simulink library "GTPR_Library"  (R2021a)
settings: Solver=VariableStepAuto  StartTime=0.0  StopTime=10.0  RelTol=1e-3
values from neighbouring files (symbols this model uses):
  aA = 0.5    [SimMechanics_GTPR_OpenLoop_CircularMotion_VS_ClosedLoop.m]
  aB = 0.5    [SimMechanics_GTPR_OpenLoop_CircularMotion_VS_ClosedLoop.m]
  aC = 0.5    [SimMechanics_GTPR_OpenLoop_CircularMotion_VS_ClosedLoop.m]
  alphaAB = deg2rad(120)    [SimMechanics_GTPR_OpenLoop_CircularMotion_VS_ClosedLoop.m]
  alphaAC = deg2rad(240)    [SimMechanics_GTPR_OpenLoop_CircularMotion_VS_ClosedLoop.m]
  eA = 0.28    [SimMechanics_GTPR_OpenLoop_CircularMotion_VS_ClosedLoop.m]
  eB = 0.28    [SimMechanics_GTPR_OpenLoop_CircularMotion_VS_ClosedLoop.m]
  eC = 0.28    [SimMechanics_GTPR_OpenLoop_CircularMotion_VS_ClosedLoop.m]
  g = -9.81    [SimMechanics_GTPR_OpenLoop_CircularMotion_VS_ClosedLoop.m]
  ILA = zeros(3)    [SimMechanics_GTPR_OpenLoop_CircularMotion_VS_ClosedLoop.m]
  IlA = zeros(3)    [SimMechanics_GTPR_OpenLoop_CircularMotion_VS_ClosedLoop.m]
  ILB = zeros(3)    [SimMechanics_GTPR_OpenLoop_CircularMotion_VS_ClosedLoop.m]
  IlB = zeros(3)    [SimMechanics_GTPR_OpenLoop_CircularMotion_VS_ClosedLoop.m]
  ILC = zeros(3)    [SimMechanics_GTPR_OpenLoop_CircularMotion_VS_ClosedLoop.m]
  IlC = zeros(3)    [SimMechanics_GTPR_OpenLoop_CircularMotion_VS_ClosedLoop.m]
  LA = 0.57    [SimMechanics_GTPR_OpenLoop_CircularMotion_VS_ClosedLoop.m]
  lA = 0.9    [SimMechanics_GTPR_OpenLoop_CircularMotion_VS_ClosedLoop.m]
  LB = 0.57    [SimMechanics_GTPR_OpenLoop_CircularMotion_VS_ClosedLoop.m]
  lB = 0.9    [SimMechanics_GTPR_OpenLoop_CircularMotion_VS_ClosedLoop.m]
  LC = 0.57    [SimMechanics_GTPR_OpenLoop_CircularMotion_VS_ClosedLoop.m]
  lC = 0.9    [SimMechanics_GTPR_OpenLoop_CircularMotion_VS_ClosedLoop.m]
  m_unaccounted = 1e-16    [SimMechanics_GTPR_OpenLoop_CircularMotion_VS_ClosedLoop.m]
  mLA = density_upperArm*VLA    (= 1.4415197891)    [SimMechanics_GTPR_OpenLoop_CircularMotion_VS_ClosedLoop.m]
  mlA = density_LowerArm*VlA    (= 0.190851753706)    [SimMechanics_GTPR_OpenLoop_CircularMotion_VS_ClosedLoop.m]
  mLB = density_upperArm*VLB    (= 1.4415197891)    [SimMechanics_GTPR_OpenLoop_CircularMotion_VS_ClosedLoop.m]
  mlB = density_LowerArm*VlB    (= 0.190851753706)    [SimMechanics_GTPR_OpenLoop_CircularMotion_VS_ClosedLoop.m]
  mLC = density_upperArm*VLC    (= 1.4415197891)    [SimMechanics_GTPR_OpenLoop_CircularMotion_VS_ClosedLoop.m]
  mlC = density_LowerArm*VlC    (= 0.190851753706)    [SimMechanics_GTPR_OpenLoop_CircularMotion_VS_ClosedLoop.m]
  mTCP = density_workTriangle * VTCP    [SimMechanics_GTPR_OpenLoop_CircularMotion_VS_ClosedLoop.m]
undefined symbols (not defined in the file or in its folder): dq1, dq2, dq3, q1, q2, q3, X, Y, Z
libraries: sm_lib x83, $bdroot x31, nesl_utility x24
(part 4 of 8)

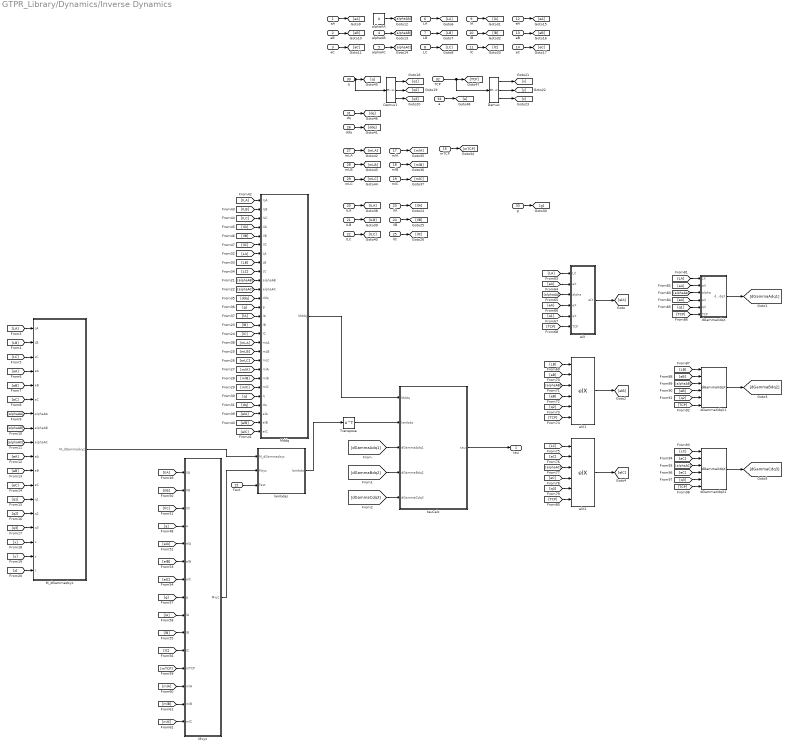
== system GTPR_Library/Dynamics/Inverse Dynamics ==
  aA : Inport
  aB : Inport  Port=2
  aC : Inport  Port=3
  alphaAB : Inport  Port=4
  alphaAC : Inport  Port=5
  LA : Inport  Port=6
  LB : Inport  Port=7
  LC : Inport  Port=8
  lA : Inport  Port=9
  lB : Inport  Port=10
  lC : Inport  Port=11
  eA : Inport  Port=12
  eB : Inport  Port=13
  eC : Inport  Port=14
  Fext : Inport  Port=15
  mTCP : Inport  Port=16
  mlA : Inport  Port=17
  mlB : Inport  Port=18
  mlC : Inport  Port=19
  ILA : Inport  Port=20
  ILB : Inport  Port=21
  ILC : Inport  Port=22
  IlA : Inport  Port=23
  IlB : Inport  Port=24
  IlC : Inport  Port=25
  ddq : Inport  Port=26
  mLA : Inport  Port=27
  mLB : Inport  Port=28
  mLC : Inport  Port=29
  q : Inport  Port=30
  dq : Inport  Port=31
  TCP : Inport  Port=32
  g : Inport  Port=33
  a : Inport  Port=34
  Demux : Demux  Outputs=3
  Demux1 : Demux  Outputs=3
  M_dGammadxyz : Subsystem
  Mddq : Subsystem
  Mxyz : Subsystem
  Transpose : Math  Operator=transpose  SaturateOnIntegerOverflow=on
  alphaAA : Constant  Value=0
  dGammaXdqX : Subsystem
  dGammaXdqX1 : $bdroot/Dynamics/Inverse Dynamics/dGammaXdqX  SystemSampleTime=-1  VariantActivationTime=update diagram  Latency=0  AutoFrameSizeCalculation=off
  dGammaXdqX2 : $bdroot/Dynamics/Inverse Dynamics/dGammaXdqX  SystemSampleTime=-1  VariantActivationTime=update diagram  Latency=0  AutoFrameSizeCalculation=off
  elX : Subsystem
  elX1 : $bdroot/Dynamics/Inverse Dynamics/elX  SystemSampleTime=-1  VariantActivationTime=update diagram  Latency=0  AutoFrameSizeCalculation=off
  elX2 : $bdroot/Dynamics/Inverse Dynamics/elX  SystemSampleTime=-1  VariantActivationTime=update diagram  Latency=0  AutoFrameSizeCalculation=off
  lambdas : MATLAB Function  TreatAsAtomicUnit=on
  tauCalc : MATLAB Function  TreatAsAtomicUnit=on
  tau : Outport
  wires:
  M_dGammadxyz/1(M_dGammadxyz) -> lambdas/1(M_dGammadxyz)
  Mxyz/1(Mxyz) -> lambdas/2(Mxyz)
  Fext/1 -> lambdas/3(Fext)
  Mddq/1(Mddq) -> tauCalc/1(Mddq)
  lambdas/1(lambda) -> Transpose/1
  elX/1(elX) -> [elA]
  dGammaXdqX/1(dGammaXdqX) -> [dGammaAdq1]
  dGammaXdqX1/1 -> [dGammaBdq2]
  elX1/1 -> [elB]
  dGammaXdqX2/1 -> [dGammaCdq3]
  elX2/1 -> [elC]
  [dGammaAdq1] -> tauCalc/3(dGammaAdq1)
  [dGammaBdq2] -> tauCalc/4(dGammaBdq2)
  [dGammaCdq3] -> tauCalc/5(dGammaCdq3)
  tauCalc/1(tau) -> tau/1
  LA/1 -> [LA]
  LB/1 -> [LB]
  LC/1 -> [LC]
  aA/1 -> [aA]
  aB/1 -> [aB]
  aC/1 -> [aC]
  alphaAA/1 -> [alphaAA]
  alphaAB/1 -> [alphaAB]
  alphaAC/1 -> [alphaAC]
  mTCP/1 -> [mTCP]
  mlA/1 -> [mlA]
  mlB/1 -> [mlB]
  mlC/1 -> [mlC]
  ILA/1 -> [ILA]
  ILB/1 -> [ILB]
  ILC/1 -> [ILC]
  ddq/1 -> [ddq]
  mLA/1 -> [mLA]
  mLB/1 -> [mLB]
  mLC/1 -> [mLC]
  q/1 -> Demux1/1, [q]
  dq/1 -> [dq]
  TCP/1 -> Demux/1, [TCP]
  lA/1 -> [lA]
  lB/1 -> [lB]
  lC/1 -> [lC]
  eC/1 -> [eC]
  eB/1 -> [eB]
  eA/1 -> [eA]
  Demux/1 -> [x]
  Demux/2 -> [y]
  Demux/3 -> [z]
  IlB/1 -> [IlB]
  g/1 -> [g]
  IlC/1 -> [IlC]
  IlA/1 -> [IlA]
  Demux1/2 -> [q2]
  Demux1/1 -> [q1]
  Demux1/3 -> [q3]
  [LA] -> M_dGammadxyz/1(LA)
  [LB] -> M_dGammadxyz/2(LB)
  [LC] -> M_dGammadxyz/3(LC)
  [aA] -> M_dGammadxyz/4(aA)
  [aB] -> M_dGammadxyz/5(aB)
  [aC] -> M_dGammadxyz/6(aC)
  [alphaAA] -> M_dGammadxyz/7(alphaAA)
  [alphaAB] -> M_dGammadxyz/8(alphaAB)
  [alphaAC] -> M_dGammadxyz/9(alphaAC)
  [eA] -> M_dGammadxyz/10(eA)
  [eB] -> M_dGammadxyz/11(eB)
  [eC] -> M_dGammadxyz/12(eC)
  [q1] -> M_dGammadxyz/13(q1)
  [q2] -> M_dGammadxyz/14(q2)
  [q3] -> M_dGammadxyz/15(q3)
  [x] -> M_dGammadxyz/16(x)
  [y] -> M_dGammadxyz/17(y)
  [z] -> M_dGammadxyz/18(z)
  [mLA] -> Mddq/17(mLA)
  [lB] -> Mddq/15(lB)
  [mLB] -> Mddq/18(mLB)
  [LA] -> Mddq/7(LA)
  [q] -> Mddq/23(q)
  [alphaAC] -> Mddq/11(alphaAC)
  [ddq] -> Mddq/12(ddq)
  [dq] -> Mddq/24(dq)
  [lC] -> Mddq/16(lC)
  [alphaAB] -> Mddq/10(alphaAB)
  [mLC] -> Mddq/19(mLC)
  [lA] -> Mddq/14(lA)
  [LB] -> Mddq/8(LB)
  [mlB] -> Mddq/21(mlB)
  [mlA] -> Mddq/20(mlA)
  [g] -> Mddq/13(g)
  [LC] -> Mddq/9(LC)
  [mlC] -> Mddq/22(mlC)
  [elA] -> Mddq/25(elA)
  [elB] -> Mddq/26(elB)
  [elC] -> Mddq/27(elC)
  [ILA] -> Mddq/1(ILA)
  [ILB] -> Mddq/2(ILB)
  [ILC] -> Mddq/3(ILC)
  [IlA] -> Mddq/4(IlA)
  [IlB] -> Mddq/5(IlB)
  [IlC] -> Mddq/6(IlC)
  [IlA] -> Mxyz/1(IlA)
  [IlB] -> Mxyz/2(IlB)
  [IlC] -> Mxyz/3(IlC)
  a/1 -> [a]
  [a] -> Mxyz/4(a)
  [elA] -> Mxyz/5(elA)
  [elC] -> Mxyz/7(elC)
  [elB] -> Mxyz/6(elB)
  [g] -> Mxyz/8(g)
  [lC] -> Mxyz/11(lC)
  [lB] -> Mxyz/10(lB)
  [lA] -> Mxyz/9(lA)
  [mTCP] -> Mxyz/12(mTCP)
  [mlA] -> Mxyz/13(mlA)
  [mlC] -> Mxyz/15(mlC)
  [mlB] -> Mxyz/14(mlB)
  [LA] -> elX/1(LX)
  [aA] -> elX/2(aX)
  [alphaAA] -> elX/3(alpha)
  [eA] -> elX/4(eX)
  [q1] -> elX/5(qX)
  [TCP] -> elX/6(TCP)
  [LB] -> elX1/1
  [alphaAB] -> elX1/3
  [q2] -> elX1/5
  [aB] -> elX1/2
  [eB] -> elX1/4
  [TCP] -> elX1/6
  [LC] -> elX2/1
  [alphaAC] -> elX2/3
  [q3] -> elX2/5
  [aC] -> elX2/2
  [eC] -> elX2/4
  [TCP] -> elX2/6
  [LA] -> dGammaXdqX/1(LX)
  [alphaAA] -> dGammaXdqX/3(alpha)
  [q1] -> dGammaXdqX/5(qX)
  [aA] -> dGammaXdqX/2(aX)
  [eA] -> dGammaXdqX/4(eX)
  [TCP] -> dGammaXdqX/6(TCP)
  [q2] -> dGammaXdqX1/5
  [alphaAB] -> dGammaXdqX1/3
  [LB] -> dGammaXdqX1/1
  [eB] -> dGammaXdqX1/4
  [aB] -> dGammaXdqX1/2
  [TCP] -> dGammaXdqX1/6
  [q3] -> dGammaXdqX2/5
  [alphaAC] -> dGammaXdqX2/3
  [LC] -> dGammaXdqX2/1
  [eC] -> dGammaXdqX2/4
  [aC] -> dGammaXdqX2/2
  [TCP] -> dGammaXdqX2/6
  Transpose/1 -> tauCalc/2(lambda)

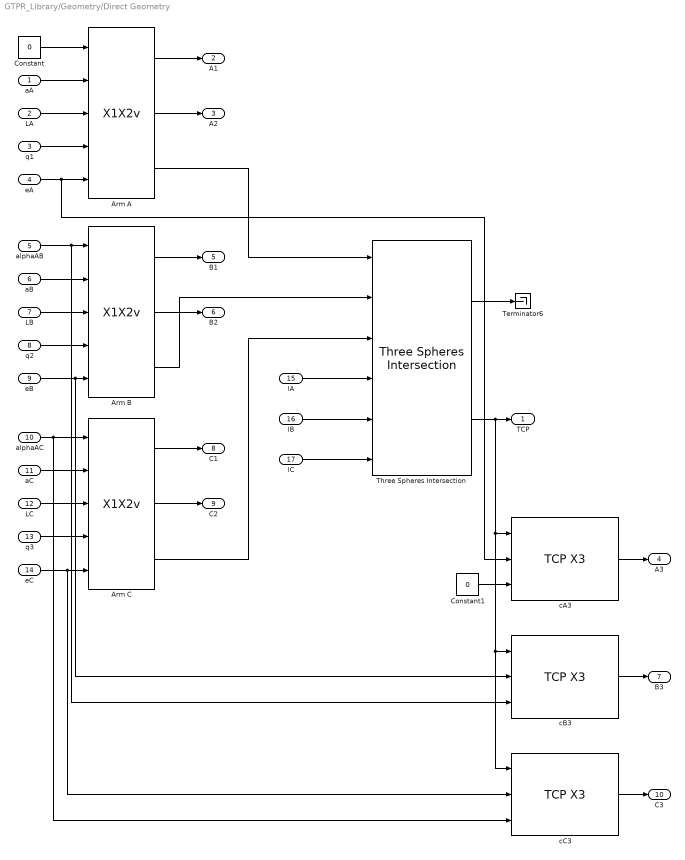
== system GTPR_Library/Geometry/Direct Geometry ==
  aA : Inport
  LA : Inport  Port=2
  q1 : Inport  Port=3
  eA : Inport  Port=4
  alphaAB : Inport  Port=5
  aB : Inport  Port=6
  LB : Inport  Port=7
  q2 : Inport  Port=8
  eB : Inport  Port=9
  alphaAC : Inport  Port=10
  aC : Inport  Port=11
  LC : Inport  Port=12
  q3 : Inport  Port=13
  eC : Inport  Port=14
  lA : Inport  Port=15
  lB : Inport  Port=16
  lC : Inport  Port=17
  Arm A : $bdroot/Other Functions/X1X2v  SystemSampleTime=-1  VariantActivationTime=update diagram  Latency=0  AutoFrameSizeCalculation=off
  Arm B : $bdroot/Other Functions/X1X2v  SystemSampleTime=-1  VariantActivationTime=update diagram  Latency=0  AutoFrameSizeCalculation=off
  Arm C : $bdroot/Other Functions/X1X2v  SystemSampleTime=-1  VariantActivationTime=update diagram  Latency=0  AutoFrameSizeCalculation=off
  Constant : Constant  Value=0
  Constant1 : Constant  Value=0
  Terminator6 : Terminator
  Three Spheres Intersection : $bdroot/Other Functions/Three Spheres Intersection  SystemSampleTime=-1  VariantActivationTime=update diagram  Latency=0  AutoFrameSizeCalculation=off
  cA3 : $bdroot/Other Functions/TCP X3  SystemSampleTime=-1  VariantActivationTime=update diagram  Latency=0  AutoFrameSizeCalculation=off
  cB3 : $bdroot/Other Functions/TCP X3  SystemSampleTime=-1  VariantActivationTime=update diagram  Latency=0  AutoFrameSizeCalculation=off
  cC3 : $bdroot/Other Functions/TCP X3  SystemSampleTime=-1  VariantActivationTime=update diagram  Latency=0  AutoFrameSizeCalculation=off
  TCP : Outport
  A1 : Outport  Port=2
  A2 : Outport  Port=3
  A3 : Outport  Port=4
  B1 : Outport  Port=5
  B2 : Outport  Port=6
  B3 : Outport  Port=7
  C1 : Outport  Port=8
  C2 : Outport  Port=9
  C3 : Outport  Port=10
  wires:
  Arm A/3 -> Three Spheres Intersection/1
  Arm C/3 -> Three Spheres Intersection/3
  Arm A/1 -> A1/1
  Arm A/2 -> A2/1
  Arm B/1 -> B1/1
  Arm B/2 -> B2/1
  Arm C/1 -> C1/1
  Arm C/2 -> C2/1
  Constant/1 -> Arm A/1
  aA/1 -> Arm A/2
  LA/1 -> Arm A/3
  q1/1 -> Arm A/4
  eA/1 -> cA3/2, Arm A/5
  alphaAB/1 -> cB3/3, Arm B/1
  aB/1 -> Arm B/2
  LB/1 -> Arm B/3
  q2/1 -> Arm B/4
  eB/1 -> cB3/2, Arm B/5
  alphaAC/1 -> cC3/3, Arm C/1
  aC/1 -> Arm C/2
  LC/1 -> Arm C/3
  q3/1 -> Arm C/4
  eC/1 -> cC3/2, Arm C/5
  Three Spheres Intersection/1 -> Terminator6/1
  Three Spheres Intersection/2 -> cC3/1, cB3/1, cA3/1, TCP/1
  lA/1 -> Three Spheres Intersection/4
  lB/1 -> Three Spheres Intersection/5
  lC/1 -> Three Spheres Intersection/6
  Arm B/3 -> Three Spheres Intersection/2
  Constant1/1 -> cA3/3
  cA3/1 -> A3/1
  cB3/1 -> B3/1
  cC3/1 -> C3/1

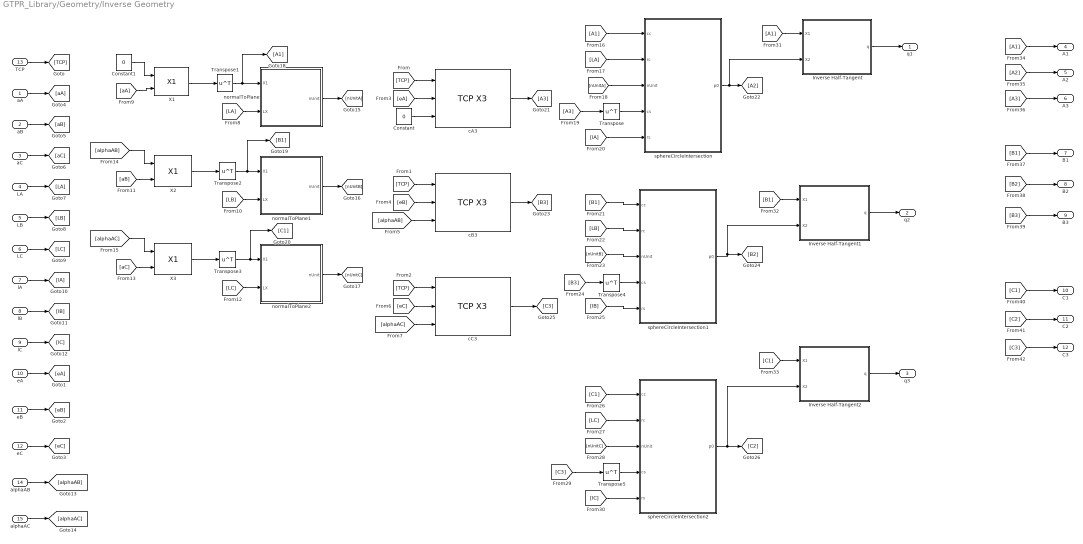
== system GTPR_Library/Geometry/Inverse Geometry ==
  aA : Inport
  aB : Inport  Port=2
  aC : Inport  Port=3
  LA : Inport  Port=4
  LB : Inport  Port=5
  LC : Inport  Port=6
  lA : Inport  Port=7
  lB : Inport  Port=8
  lC : Inport  Port=9
  eA : Inport  Port=10
  eB : Inport  Port=11
  eC : Inport  Port=12
  TCP : Inport  Port=13
  alphaAB : Inport  Port=14
  alphaAC : Inport  Port=15
  Constant : Constant  Value=0
  Constant1 : Constant  Value=0
  Inverse Half-Tangent : MATLAB Function  TreatAsAtomicUnit=on
  Inverse Half-Tangent1 : MATLAB Function  TreatAsAtomicUnit=on
  Inverse Half-Tangent2 : MATLAB Function  TreatAsAtomicUnit=on
  Transpose{,1..5} (6 alike) : Math  Operator=transpose  SaturateOnIntegerOverflow=on
  X1 : $bdroot/Other Functions/X1  SystemSampleTime=-1  VariantActivationTime=update diagram  Latency=0  AutoFrameSizeCalculation=off
  X2 : $bdroot/Other Functions/X1  SystemSampleTime=-1  VariantActivationTime=update diagram  Latency=0  AutoFrameSizeCalculation=off
  X3 : $bdroot/Other Functions/X1  SystemSampleTime=-1  VariantActivationTime=update diagram  Latency=0  AutoFrameSizeCalculation=off
  cA3 : $bdroot/Other Functions/TCP X3  SystemSampleTime=-1  VariantActivationTime=update diagram  Latency=0  AutoFrameSizeCalculation=off
  cB3 : $bdroot/Other Functions/TCP X3  SystemSampleTime=-1  VariantActivationTime=update diagram  Latency=0  AutoFrameSizeCalculation=off
  cC3 : $bdroot/Other Functions/TCP X3  SystemSampleTime=-1  VariantActivationTime=update diagram  Latency=0  AutoFrameSizeCalculation=off
  normalToPlane : MATLAB Function  TreatAsAtomicUnit=on
  normalToPlane1 : MATLAB Function  TreatAsAtomicUnit=on
  normalToPlane2 : MATLAB Function  TreatAsAtomicUnit=on
  sphereCircleIntersection : MATLAB Function  TreatAsAtomicUnit=on
  sphereCircleIntersection1 : MATLAB Function  TreatAsAtomicUnit=on
  sphereCircleIntersection2 : MATLAB Function  TreatAsAtomicUnit=on
  q1 : Outport
  q2 : Outport  Port=2
  q3 : Outport  Port=3
  A1 : Outport  Port=4
  A2 : Outport  Port=5
  A3 : Outport  Port=6
  B1 : Outport  Port=7
  B2 : Outport  Port=8
  B3 : Outport  Port=9
  C1 : Outport  Port=10
  C2 : Outport  Port=11
  C3 : Outport  Port=12
  wires:
  TCP/1 -> [TCP]
  [TCP] -> cA3/1
  Constant/1 -> cA3/3
  [TCP] -> cB3/1
  [eB] -> cB3/2
  [alphaAB] -> cB3/3
  [TCP] -> cC3/1
  [eC] -> cC3/2
  eB/1 -> [eB]
  eC/1 -> [eC]
  eA/1 -> [eA]
  aA/1 -> [aA]
  aB/1 -> [aB]
  aC/1 -> [aC]
  LA/1 -> [LA]
  LB/1 -> [LB]
  LC/1 -> [LC]
  lA/1 -> [lA]
  lC/1 -> [lC]
  lB/1 -> [lB]
  alphaAB/1 -> [alphaAB]
  [eA] -> cA3/2
  alphaAC/1 -> [alphaAC]
  [alphaAC] -> cC3/3
  [LA] -> normalToPlane/2(LX)
  Constant1/1 -> X1/1
  [aA] -> X1/2
  normalToPlane/1(nUnit) -> [nUnitA]
  normalToPlane1/1(nUnit) -> [nUnitB]
  [aB] -> X2/2
  [LB] -> normalToPlane1/2(LX)
  [alphaAB] -> X2/1
  normalToPlane2/1(nUnit) -> [nUnitC]
  [aC] -> X3/2
  [LC] -> normalToPlane2/2(LX)
  [alphaAC] -> X3/1
  [A1] -> sphereCircleIntersection/1(cc)
  [LA] -> sphereCircleIntersection/2(rc)
  cA3/1 -> [A3]
  [A3] -> Transpose/1
  [lA] -> sphereCircleIntersection/5(rs)
  sphereCircleIntersection/1(p0) -> Inverse Half-Tangent/2(X2), [A2]
  [lC] -> sphereCircleIntersection2/5(rs)
  [LC] -> sphereCircleIntersection2/2(rc)
  [nUnitC] -> sphereCircleIntersection2/3(nUnit)
  [C1] -> sphereCircleIntersection2/1(cc)
  [C3] -> Transpose5/1
  cC3/1 -> [C3]
  cB3/1 -> [B3]
  [A1] -> Inverse Half-Tangent/1(X1)
  Inverse Half-Tangent/1(q) -> q1/1
  [B1] -> Inverse Half-Tangent1/1(X1)
  sphereCircleIntersection1/1(p0) -> Inverse Half-Tangent1/2(X2), [B2]
  Inverse Half-Tangent1/1(q) -> q2/1
  [C1] -> Inverse Half-Tangent2/1(X1)
  sphereCircleIntersection2/1(p0) -> Inverse Half-Tangent2/2(X2), [C2]
  Inverse Half-Tangent2/1(q) -> q3/1
  [A1] -> A1/1
  [A2] -> A2/1
  [A3] -> A3/1
  [B1] -> B1/1
  [B2] -> B2/1
  [B3] -> B3/1
  [C1] -> C1/1
  [C2] -> C2/1
  [C3] -> C3/1
  X1/1 -> Transpose1/1
  Transpose1/1 -> [A1], normalToPlane/1(X1)
  X2/1 -> Transpose2/1
  Transpose2/1 -> [B1], normalToPlane1/1(X1)
  X3/1 -> Transpose3/1
  Transpose3/1 -> [C1], normalToPlane2/1(X1)
  [B1] -> sphereCircleIntersection1/1(cc)
  [LB] -> sphereCircleIntersection1/2(rc)
  [nUnitB] -> sphereCircleIntersection1/3(nUnit)
  [B3] -> Transpose4/1
  [lB] -> sphereCircleIntersection1/5(rs)
  Transpose/1 -> sphereCircleIntersection/4(cs)
  [nUnitA] -> sphereCircleIntersection/3(nUnit)
  Transpose4/1 -> sphereCircleIntersection1/4(cs)
  Transpose5/1 -> sphereCircleIntersection2/4(cs)

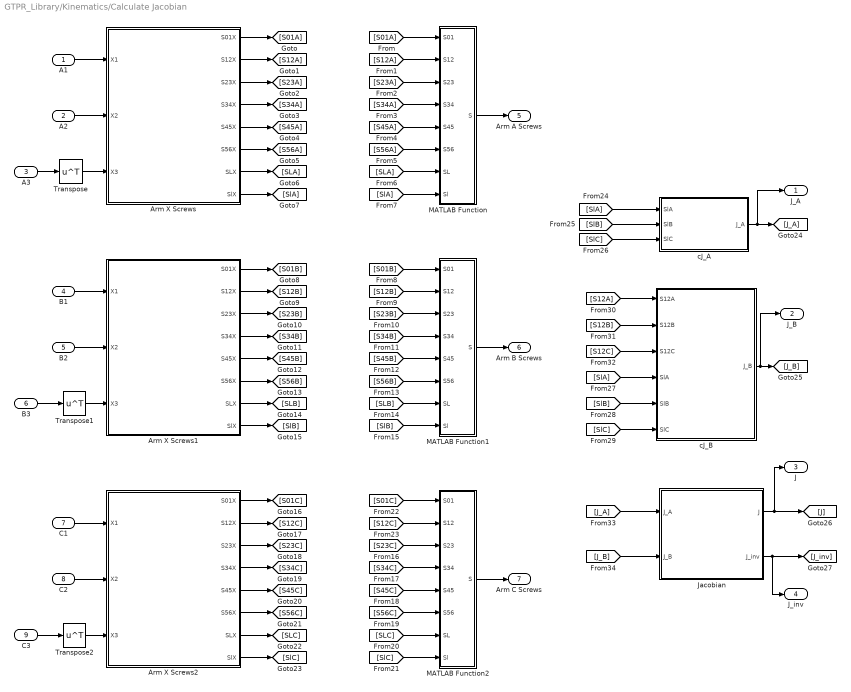
== system GTPR_Library/Kinematics/Calculate Jacobian ==
  A1 : Inport
  A2 : Inport  Port=2
  A3 : Inport  Port=3
  B1 : Inport  Port=4
  B2 : Inport  Port=5
  B3 : Inport  Port=6
  C1 : Inport  Port=7
  C2 : Inport  Port=8
  C3 : Inport  Port=9
  Arm X Screws : MATLAB Function  TreatAsAtomicUnit=on
  Arm X Screws1 : MATLAB Function  TreatAsAtomicUnit=on
  Arm X Screws2 : MATLAB Function  TreatAsAtomicUnit=on
  Jacobian : MATLAB Function  TreatAsAtomicUnit=on
  MATLAB Function : MATLAB Function  TreatAsAtomicUnit=on
  MATLAB Function1 : MATLAB Function  TreatAsAtomicUnit=on
  MATLAB Function2 : MATLAB Function  TreatAsAtomicUnit=on
  Transpose : Math  Operator=transpose  SaturateOnIntegerOverflow=on
  Transpose1 : Math  Operator=transpose  SaturateOnIntegerOverflow=on
  Transpose2 : Math  Operator=transpose  SaturateOnIntegerOverflow=on
  cJ_A : MATLAB Function  TreatAsAtomicUnit=on
  cJ_B : MATLAB Function  TreatAsAtomicUnit=on
  J_A : Outport
  J_B : Outport  Port=2
  J : Outport  Port=3
  J_inv : Outport  Port=4
  Arm A Screws : Outport  Port=5
  Arm B Screws : Outport  Port=6
  Arm C Screws : Outport  Port=7
  wires:
  A1/1 -> Arm X Screws/1(X1)
  A2/1 -> Arm X Screws/2(X2)
  A3/1 -> Transpose/1
  Arm X Screws/1(S01X) -> [S01A]
  Arm X Screws/2(S12X) -> [S12A]
  Arm X Screws/3(S23X) -> [S23A]
  Arm X Screws/4(S34X) -> [S34A]
  Arm X Screws/5(S45X) -> [S45A]
  Arm X Screws/6(S56X) -> [S56A]
  Arm X Screws/7(SLX) -> [SLA]
  Arm X Screws/8(SlX) -> [SlA]
  [S01A] -> MATLAB Function/1(S01)
  [S12A] -> MATLAB Function/2(S12)
  [S23A] -> MATLAB Function/3(S23)
  [S34A] -> MATLAB Function/4(S34)
  [S45A] -> MATLAB Function/5(S45)
  [S56A] -> MATLAB Function/6(S56)
  [SLA] -> MATLAB Function/7(SL)
  [SlA] -> MATLAB Function/8(Sl)
  Arm X Screws1/2(S12X) -> [S12B]
  B2/1 -> Arm X Screws1/2(X2)
  B3/1 -> Transpose1/1
  B1/1 -> Arm X Screws1/1(X1)
  Arm X Screws1/3(S23X) -> [S23B]
  Arm X Screws1/6(S56X) -> [S56B]
  Arm X Screws1/8(SlX) -> [SlB]
  Arm X Screws1/4(S34X) -> [S34B]
  Arm X Screws1/5(S45X) -> [S45B]
  Arm X Screws1/1(S01X) -> [S01B]
  Arm X Screws1/7(SLX) -> [SLB]
  Arm X Screws2/2(S12X) -> [S12C]
  C2/1 -> Arm X Screws2/2(X2)
  C3/1 -> Transpose2/1
  C1/1 -> Arm X Screws2/1(X1)
  Arm X Screws2/3(S23X) -> [S23C]
  Arm X Screws2/6(S56X) -> [S56C]
  Arm X Screws2/8(SlX) -> [SlC]
  Arm X Screws2/4(S34X) -> [S34C]
  Arm X Screws2/5(S45X) -> [S45C]
  Arm X Screws2/1(S01X) -> [S01C]
  Arm X Screws2/7(SLX) -> [SLC]
  [S45B] -> MATLAB Function1/5(S45)
  [S23B] -> MATLAB Function1/3(S23)
  [S01B] -> MATLAB Function1/1(S01)
  [SlB] -> MATLAB Function1/8(Sl)
  [S12B] -> MATLAB Function1/2(S12)
  [SLB] -> MATLAB Function1/7(SL)
  [S34B] -> MATLAB Function1/4(S34)
  [S56B] -> MATLAB Function1/6(S56)
  [S12C] -> MATLAB Function2/2(S12)
  [S23C] -> MATLAB Function2/3(S23)
  [S01C] -> MATLAB Function2/1(S01)
  [S34C] -> MATLAB Function2/4(S34)
  [SLC] -> MATLAB Function2/7(SL)
  [S45C] -> MATLAB Function2/5(S45)
  [S56C] -> MATLAB Function2/6(S56)
  [SlC] -> MATLAB Function2/8(Sl)
  [SlA] -> cJ_A/1(SlA)
  [SlB] -> cJ_A/2(SlB)
  [SlC] -> cJ_A/3(SlC)
  cJ_A/1(J_A) -> J_A/1, [J_A]
  [SlB] -> cJ_B/5(SlB)
  [SlA] -> cJ_B/4(SlA)
  [SlC] -> cJ_B/6(SlC)
  [S12A] -> cJ_B/1(S12A)
  [S12B] -> cJ_B/2(S12B)
  [S12C] -> cJ_B/3(S12C)
  cJ_B/1(J_B) -> J_B/1, [J_B]
  [J_A] -> Jacobian/1(J_A)
  [J_B] -> Jacobian/2(J_B)
  Jacobian/1(J) -> J/1, [J]
  Jacobian/2(J_inv) -> J_inv/1, [J_inv]
  MATLAB Function/1(S) -> Arm A Screws/1
  MATLAB Function1/1(S) -> Arm B Screws/1
  MATLAB Function2/1(S) -> Arm C Screws/1
  Transpose/1 -> Arm X Screws/3(X3)
  Transpose1/1 -> Arm X Screws1/3(X3)
  Transpose2/1 -> Arm X Screws2/3(X3)

== system GTPR_Library/Kinematics/Direct Kinematics ==
  A1 : Inport
  A2 : Inport  Port=2
  A3 : Inport  Port=3
  B1 : Inport  Port=4
  B2 : Inport  Port=5
  B3 : Inport  Port=6
  C1 : Inport  Port=7
  C2 : Inport  Port=8
  C3 : Inport  Port=9
  dq : Inport  Port=10
  Calculate Jacobian : $bdroot/Kinematics/Calculate Jacobian  SystemSampleTime=-1  VariantActivationTime=update diagram  Latency=0  AutoFrameSizeCalculation=off
  Product : Product
  Terminator{,1..5} (6 alike) : Terminator
  v : Outport
  wires:
  A1/1 -> Calculate Jacobian/1
  A2/1 -> Calculate Jacobian/2
  A3/1 -> Calculate Jacobian/3
  B1/1 -> Calculate Jacobian/4
  B2/1 -> Calculate Jacobian/5
  B3/1 -> Calculate Jacobian/6
  C1/1 -> Calculate Jacobian/7
  C2/1 -> Calculate Jacobian/8
  C3/1 -> Calculate Jacobian/9
  dq/1 -> Product/2
  Calculate Jacobian/1 -> Terminator/1
  Calculate Jacobian/2 -> Terminator1/1
  Calculate Jacobian/4 -> Terminator2/1
  Calculate Jacobian/5 -> Terminator3/1
  Calculate Jacobian/6 -> Terminator4/1
  Calculate Jacobian/7 -> Terminator5/1
  Calculate Jacobian/3 -> Product/1
  Product/1 -> v/1

== system GTPR_Library/Kinematics/Direct Kinematics Acceleration ==
  A1 : Inport
  A2 : Inport  Port=2
  A3 : Inport  Port=3
  B1 : Inport  Port=4
  B2 : Inport  Port=5
  B3 : Inport  Port=6
  C1 : Inport  Port=7
  C2 : Inport  Port=8
  C3 : Inport  Port=9
  ddq : Inport  Port=10
  Calculate Jacobian : $bdroot/Kinematics/Calculate Jacobian  SystemSampleTime=-1  VariantActivationTime=update diagram  Latency=0  AutoFrameSizeCalculation=off
  Jacobian_C : MATLAB Function  TreatAsAtomicUnit=on
  Terminator2 : Terminator
  Terminator3 : Terminator
  directKinematics_Acceleration : MATLAB Function  TreatAsAtomicUnit=on
  a : Outport
  wires:
  A1/1 -> Calculate Jacobian/1
  C1/1 -> Calculate Jacobian/7
  Calculate Jacobian/4 -> Terminator2/1
  Calculate Jacobian/2 -> directKinematics_Acceleration/3(J_B)
  B3/1 -> Calculate Jacobian/6
  B1/1 -> Calculate Jacobian/4
  A2/1 -> Calculate Jacobian/2
  C2/1 -> Calculate Jacobian/8
  Calculate Jacobian/1 -> directKinematics_Acceleration/2(J_A)
  B2/1 -> Calculate Jacobian/5
  A3/1 -> Calculate Jacobian/3
  C3/1 -> Calculate Jacobian/9
  Calculate Jacobian/3 -> Terminator3/1
  directKinematics_Acceleration/1(a) -> a/1
  Calculate Jacobian/5 -> Jacobian_C/1(ScrewsArm_A)
  Calculate Jacobian/6 -> Jacobian_C/2(ScrewsArm_B)
  Calculate Jacobian/7 -> Jacobian_C/3(ScrewsArm_C)
  Jacobian_C/1(J_C) -> directKinematics_Acceleration/4(J_C)
  ddq/1 -> directKinematics_Acceleration/1(ddq)

== system GTPR_Library/Kinematics/Inverse Kinematics ==
  A1 : Inport
  A2 : Inport  Port=2
  A3 : Inport  Port=3
  B1 : Inport  Port=4
  B2 : Inport  Port=5
  B3 : Inport  Port=6
  C1 : Inport  Port=7
  C2 : Inport  Port=8
  C3 : Inport  Port=9
  v : Inport  Port=10
  Calculate Jacobian : $bdroot/Kinematics/Calculate Jacobian  SystemSampleTime=-1  VariantActivationTime=update diagram  Latency=0  AutoFrameSizeCalculation=off
  Product : Product  Multiplication=Matrix(*)
  Terminator{,1..5} (6 alike) : Terminator
  dq : Outport
  wires:
  A1/1 -> Calculate Jacobian/1
  C1/1 -> Calculate Jacobian/7
  Calculate Jacobian/6 -> Terminator4/1
  Calculate Jacobian/4 -> Product/1
  Calculate Jacobian/2 -> Terminator1/1
  B3/1 -> Calculate Jacobian/6
  B1/1 -> Calculate Jacobian/4
  A2/1 -> Calculate Jacobian/2
  C2/1 -> Calculate Jacobian/8
  Calculate Jacobian/7 -> Terminator5/1
  Calculate Jacobian/1 -> Terminator/1
  B2/1 -> Calculate Jacobian/5
  Calculate Jacobian/5 -> Terminator3/1
  v/1 -> Product/2
  A3/1 -> Calculate Jacobian/3
  Product/1 -> dq/1
  C3/1 -> Calculate Jacobian/9
  Calculate Jacobian/3 -> Terminator2/1

== system GTPR_Library/Kinematics/Inverse Kinematics Acceleration ==
  A1 : Inport
  A2 : Inport  Port=2
  A3 : Inport  Port=3
  B1 : Inport  Port=4
  B2 : Inport  Port=5
  B3 : Inport  Port=6
  C1 : Inport  Port=7
  C2 : Inport  Port=8
  C3 : Inport  Port=9
  v : Inport  Port=10
  a : Inport  Port=11
  Calculate Jacobian : $bdroot/Kinematics/Calculate Jacobian  SystemSampleTime=-1  VariantActivationTime=update diagram  Latency=0  AutoFrameSizeCalculation=off
  Jacobian_C : MATLAB Function  TreatAsAtomicUnit=on
  Terminator2 : Terminator
  Terminator3 : Terminator
  inverseKinematics_Acceleration : MATLAB Function  TreatAsAtomicUnit=on
  ddq : Outport
  wires:
  a/1 -> inverseKinematics_Acceleration/1(a)
  Calculate Jacobian/1 -> inverseKinematics_Acceleration/2(J_A)
  Calculate Jacobian/2 -> inverseKinematics_Acceleration/3(J_B)
  Calculate Jacobian/6 -> Jacobian_C/2(ScrewsArm_B)
  Jacobian_C/1(J_C) -> inverseKinematics_Acceleration/4(J_C)
  A2/1 -> Calculate Jacobian/2
  C2/1 -> Calculate Jacobian/8
  B1/1 -> Calculate Jacobian/4
  B2/1 -> Calculate Jacobian/5
  B3/1 -> Calculate Jacobian/6
  Calculate Jacobian/4 -> Terminator2/1
  A1/1 -> Calculate Jacobian/1
  Calculate Jacobian/3 -> Terminator3/1
  A3/1 -> Calculate Jacobian/3
  C3/1 -> Calculate Jacobian/9
  C1/1 -> Calculate Jacobian/7
  inverseKinematics_Acceleration/1(ddq) -> ddq/1
  Calculate Jacobian/5 -> Jacobian_C/1(ScrewsArm_A)
  Calculate Jacobian/7 -> Jacobian_C/3(ScrewsArm_C)
  v/1 -> Jacobian_C/4(v)

== system GTPR_Library/Other Functions/TCP X3 ==
  TCP : Inport
  eX : Inport  Port=2
  alpha : Inport  Port=3
  Add : Sum  Inputs=+-
  Constant : Constant  Value=0
  Mux : Mux  Inputs=3
  Product : Product  Multiplication=Matrix(*)
  Rz : MATLAB Function  TreatAsAtomicUnit=on
  Transpose : Math  Operator=transpose  SaturateOnIntegerOverflow=on
  Transpose1 : Math  Operator=transpose  SaturateOnIntegerOverflow=on
  Transpose2 : Math  Operator=transpose  SaturateOnIntegerOverflow=on
  X3 : Outport
  wires:
  alpha/1 -> Rz/1(theta)
  Rz/1(R) -> Transpose/1
  Transpose/1 -> Product/2
  eX/1 -> Mux/2
  Constant/1 -> Mux/3, Mux/1
  Product/1 -> Add/2
  Add/1 -> X3/1
  Mux/1 -> Transpose1/1
  Transpose1/1 -> Product/1
  TCP/1 -> Transpose2/1
  Transpose2/1 -> Add/1

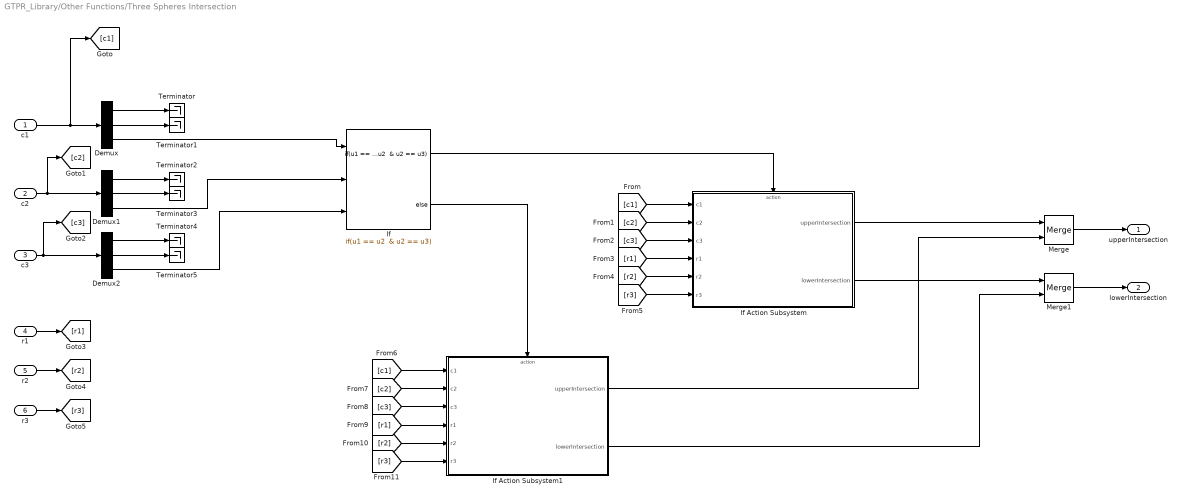
== system GTPR_Library/Other Functions/Three Spheres Intersection ==
  c1 : Inport
  c2 : Inport  Port=2
  c3 : Inport  Port=3
  r1 : Inport  Port=4
  r2 : Inport  Port=5
  r3 : Inport  Port=6
  Demux : Demux  Outputs=3
  Demux1 : Demux  Outputs=3
  Demux2 : Demux  Outputs=3
  If : If  NumInputs=3  IfExpression="u1 == u2  & u2 == u3"
  If Action Subsystem : Subsystem  TreatAsAtomicUnit=on
  If Action Subsystem1 : Subsystem  TreatAsAtomicUnit=on
  Merge : Merge
  Merge1 : Merge
  Terminator{,1..5} (6 alike) : Terminator
  upperIntersection : Outport
  lowerIntersection : Outport  Port=2
  wires:
  c1/1 -> [c1], Demux/1
  c2/1 -> [c2], Demux1/1
  c3/1 -> [c3], Demux2/1
  Demux/3 -> If/1
  Demux1/3 -> If/2
  Demux2/3 -> If/3
  Demux/1 -> Terminator/1
  Demux/2 -> Terminator1/1
  Demux1/1 -> Terminator2/1
  Demux1/2 -> Terminator3/1
  Demux2/1 -> Terminator4/1
  Demux2/2 -> Terminator5/1
  If/1 -> If Action Subsystem/Action
  [c1] -> If Action Subsystem/1(c1)
  r1/1 -> [r1]
  r2/1 -> [r2]
  r3/1 -> [r3]
  [c2] -> If Action Subsystem/2(c2)
  [c3] -> If Action Subsystem/3(c3)
  [r1] -> If Action Subsystem/4(r1)
  [r2] -> If Action Subsystem/5(r2)
  [r3] -> If Action Subsystem/6(r3)
  If Action Subsystem/1(upperIntersection) -> Merge/1
  If Action Subsystem/2(lowerIntersection) -> Merge1/1
  [c2] -> If Action Subsystem1/2(c2)
  [r1] -> If Action Subsystem1/4(r1)
  [r3] -> If Action Subsystem1/6(r3)
  [c1] -> If Action Subsystem1/1(c1)
  [c3] -> If Action Subsystem1/3(c3)
  [r2] -> If Action Subsystem1/5(r2)
  If/2 -> If Action Subsystem1/Action
  If Action Subsystem1/1(upperIntersection) -> Merge/2
  If Action Subsystem1/2(lowerIntersection) -> Merge1/2
  Merge/1 -> upperIntersection/1
  Merge1/1 -> lowerIntersection/1

== system GTPR_Library/Other Functions/X1 ==
  alpha : Inport
  aX : Inport  Port=2
  Constant : Constant  Value=0
  Constant1 : Constant  Value=0
  Gain : Gain  Gain=-1
  Mux : Mux  Inputs=3
  Product : Product  Multiplication=Matrix(*)
  Rz1 : MATLAB Function  TreatAsAtomicUnit=on
  Transpose : Math  Operator=transpose  SaturateOnIntegerOverflow=on
  Transpose1 : Math  Operator=transpose  SaturateOnIntegerOverflow=on
  X1 : Outport
  wires:
  alpha/1 -> Rz1/1(theta)
  Mux/1 -> Transpose1/1
  Rz1/1(R) -> Transpose/1
  Product/1 -> X1/1
  Constant/1 -> Mux/1
  Constant1/1 -> Mux/3
  Gain/1 -> Mux/2
  aX/1 -> Gain/1
  Transpose1/1 -> Product/1
  Transpose/1 -> Product/2

== system GTPR_Library/Other Functions/X1X2 ==
  alpha : Inport
  aX : Inport  Port=2
  LX : Inport  Port=3
  qX : Inport  Port=4
  X1 : $bdroot/Other Functions/X1  SystemSampleTime=-1  VariantActivationTime=update diagram  Latency=0  AutoFrameSizeCalculation=off
  X2 : $bdroot/Other Functions/X2  SystemSampleTime=-1  VariantActivationTime=update diagram  Latency=0  AutoFrameSizeCalculation=off
  x1 : Outport
  x2 : Outport  Port=2
  wires:
  alpha/1 -> X2/2, X1/1
  X1/1 -> X2/1, x1/1
  LX/1 -> X2/3
  aX/1 -> X1/2
  X2/1 -> x2/1
  qX/1 -> X2/4

== system GTPR_Library/Other Functions/X1X2v ==
  alpha : Inport
  aX : Inport  Port=2
  LX : Inport  Port=3
  qX : Inport  Port=4
  eX : Inport  Port=5
  X1X2 : $bdroot/Geometry/X1X2  SystemSampleTime=-1  VariantActivationTime=update diagram  Latency=0  AutoFrameSizeCalculation=off
  X2v : $bdroot/Other Functions/X2v  SystemSampleTime=-1  VariantActivationTime=update diagram  Latency=0  AutoFrameSizeCalculation=off
  x1 : Outport
  x2 : Outport  Port=2
  x2v : Outport  Port=3
  wires:
  X1X2/2 -> x2/1, X2v/1
  alpha/1 -> X2v/2, X1X2/1
  eX/1 -> X2v/3
  qX/1 -> X1X2/4
  LX/1 -> X1X2/3
  aX/1 -> X1X2/2
  X1X2/1 -> x1/1
  X2v/1 -> x2v/1

== system GTPR_Library/Other Functions/X2 ==
  X1 : Inport
  alpha : Inport  Port=2
  LX : Inport  Port=3
  qX : Inport  Port=4
  Add : Sum
  Constant : Constant  Value=0
  Cos : Trigonometry  Operator=cos
  Gain : Gain  Gain=-1
  Mux : Mux  Inputs=3
  Product : Product
  Product1 : Product
  Rz : MATLAB Function  TreatAsAtomicUnit=on
  Sin : Trigonometry
  Transpose : Math  Operator=transpose  SaturateOnIntegerOverflow=on
  X2 : Outport
  wires:
  alpha/1 -> Rz/1(theta)
  Rz/1(R) -> Transpose/1
  qX/1 -> Gain/1
  Gain/1 -> Sin/1, Cos/1
  Cos/1 -> Mux/2
  Sin/1 -> Mux/3
  Constant/1 -> Mux/1
  Transpose/1 -> Product/1
  LX/1 -> Product/2
  Product/1 -> Product1/1
  Mux/1 -> Product1/2
  X1/1 -> Add/1
  Product1/1 -> Add/2
  Add/1 -> X2/1

== system GTPR_Library/Other Functions/X2v ==
  X2 : Inport
  alpha : Inport  Port=2
  eX : Inport  Port=3
  Add : Sum  Inputs=+-
  Constant : Constant  Value=0
  Mux : Mux  Inputs=3
  Product : Product
  Rz : MATLAB Function  TreatAsAtomicUnit=on
  Transpose : Math  Operator=transpose  SaturateOnIntegerOverflow=on
  X2v : Outport
  wires:
  X2/1 -> Add/1
  Add/1 -> X2v/1
  alpha/1 -> Rz/1(theta)
  Rz/1(R) -> Transpose/1
  eX/1 -> Mux/2
  Constant/1 -> Mux/3, Mux/1
  Mux/1 -> Product/2
  Transpose/1 -> Product/1
  Product/1 -> Add/2

== system GTPR_Library/Dynamics/Initialize Dynamic Equations/If Action Subsystem ==
  Action Port : ActionPort  ActionPortLabel=if(u1 == 0)
  Initialize Dynamics : MATLAB Function  TreatAsAtomicUnit=on
  String Constant : StringConstant  String=filepath
  wires:
  String Constant/1 -> Initialize Dynamics/1(filepath)

== system GTPR_Library/Dynamics/Inverse Dynamics/M_dGammadxyz ==
  LA : Inport
  LB : Inport  Port=2
  LC : Inport  Port=3
  aA : Inport  Port=4
  aB : Inport  Port=5
  aC : Inport  Port=6
  alphaAA : Inport  Port=7
  alphaAB : Inport  Port=8
  alphaAC : Inport  Port=9
  eA : Inport  Port=10
  eB : Inport  Port=11
  eC : Inport  Port=12
  q1 : Inport  Port=13
  q2 : Inport  Port=14
  q3 : Inport  Port=15
  x : Inport  Port=16
  y : Inport  Port=17
  z : Inport  Port=18
  Interpreted MATLAB Function : MATLABFcn  MATLABFcn=obj.M_dGammadxyzf
  Mux : Mux  Inputs=18
  M_dGammadxyz : Outport
  wires:
  Interpreted MATLAB Function/1 -> M_dGammadxyz/1
  aA/1 -> Mux/4
  q3/1 -> Mux/15
  aC/1 -> Mux/6
  x/1 -> Mux/16
  eA/1 -> Mux/10
  Mux/1 -> Interpreted MATLAB Function/1
  eC/1 -> Mux/12
  z/1 -> Mux/18
  alphaAC/1 -> Mux/9
  LA/1 -> Mux/1
  y/1 -> Mux/17
  q2/1 -> Mux/14
  LB/1 -> Mux/2
  alphaAA/1 -> Mux/7
  aB/1 -> Mux/5
  alphaAB/1 -> Mux/8
  LC/1 -> Mux/3
  eB/1 -> Mux/11
  q1/1 -> Mux/13

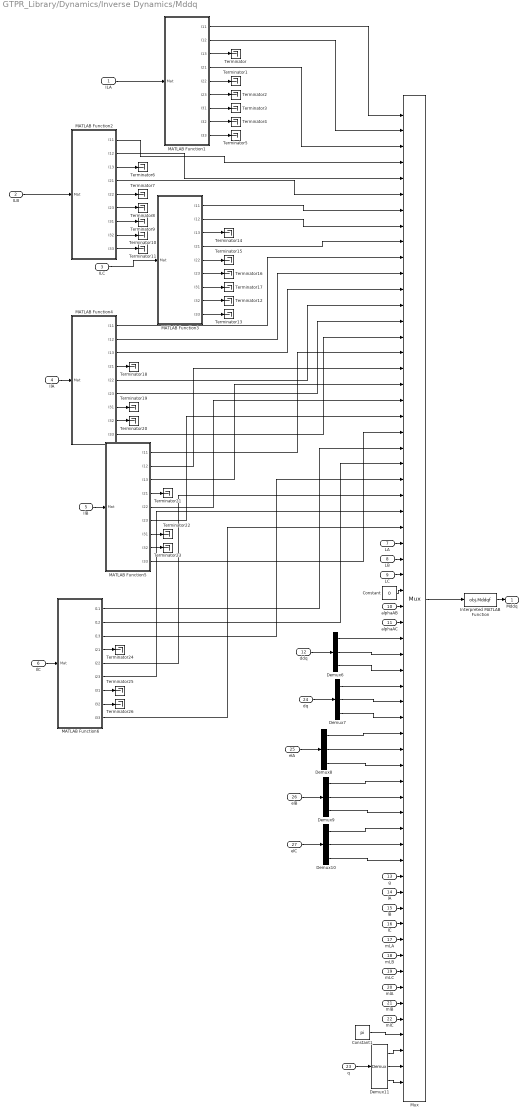
== system GTPR_Library/Dynamics/Inverse Dynamics/Mddq ==
  ILA : Inport
  ILB : Inport  Port=2
  ILC : Inport  Port=3
  IlA : Inport  Port=4
  IlB : Inport  Port=5
  IlC : Inport  Port=6
  LA : Inport  Port=7
  LB : Inport  Port=8
  LC : Inport  Port=9
  alphaAB : Inport  Port=10
  alphaAC : Inport  Port=11
  ddq : Inport  Port=12
  g : Inport  Port=13
  lA : Inport  Port=14
  lB : Inport  Port=15
  lC : Inport  Port=16
  mLA : Inport  Port=17
  mLB : Inport  Port=18
  mLC : Inport  Port=19
  mlA : Inport  Port=20
  mlB : Inport  Port=21
  mlC : Inport  Port=22
  q : Inport  Port=23
  dq : Inport  Port=24
  elA : Inport  Port=25
  elB : Inport  Port=26
  elC : Inport  Port=27
  Constant : Constant  Value=0
  Constant1 : Constant  Value=pi
  Demux{6..11} (6 alike) : Demux  Outputs=3
  Interpreted MATLAB Function : MATLABFcn  MATLABFcn=obj.Mddqf
  MATLAB Function1 : MATLAB Function  TreatAsAtomicUnit=on
  MATLAB Function2 : MATLAB Function  TreatAsAtomicUnit=on
  MATLAB Function3 : MATLAB Function  TreatAsAtomicUnit=on
  MATLAB Function4 : MATLAB Function  TreatAsAtomicUnit=on
  MATLAB Function5 : MATLAB Function  TreatAsAtomicUnit=on
  MATLAB Function6 : MATLAB Function  TreatAsAtomicUnit=on
  Mux : Mux  Inputs=62
  Terminator{,1..26} (27 alike) : Terminator
  Mddq : Outport
  wires:
  Mux/1 -> Interpreted MATLAB Function/1
  LB/1 -> Mux/29
  Interpreted MATLAB Function/1 -> Mddq/1
  LA/1 -> Mux/28
  MATLAB Function1/1(I11) -> Mux/1
  MATLAB Function1/2(I12) -> Mux/2
  MATLAB Function1/4(I21) -> Mux/3
  MATLAB Function1/3(I13) -> Terminator/1
  MATLAB Function1/5(I22) -> Terminator1/1
  MATLAB Function1/6(I23) -> Terminator2/1
  MATLAB Function1/7(I31) -> Terminator3/1
  MATLAB Function1/8(I32) -> Terminator4/1
  MATLAB Function1/9(I33) -> Terminator5/1
  ILA/1 -> MATLAB Function1/1(Mat)
  MATLAB Function2/2(I12) -> Mux/5
  MATLAB Function2/5(I22) -> Terminator7/1
  MATLAB Function2/6(I23) -> Terminator8/1
  MATLAB Function2/9(I33) -> Terminator11/1
  MATLAB Function2/1(I11) -> Mux/4
  MATLAB Function2/8(I32) -> Terminator10/1
  MATLAB Function2/7(I31) -> Terminator9/1
  MATLAB Function2/3(I13) -> Terminator6/1
  ILB/1 -> MATLAB Function2/1(Mat)
  MATLAB Function2/4(I21) -> Mux/6
  MATLAB Function3/4(I21) -> Mux/9
  MATLAB Function3/1(I11) -> Mux/7
  MATLAB Function3/8(I32) -> Terminator12/1
  ILC/1 -> MATLAB Function3/1(Mat)
  MATLAB Function3/3(I13) -> Terminator14/1
  MATLAB Function3/7(I31) -> Terminator17/1
  MATLAB Function3/6(I23) -> Terminator16/1
  MATLAB Function3/5(I22) -> Terminator15/1
  MATLAB Function3/9(I33) -> Terminator13/1
  MATLAB Function3/2(I12) -> Mux/8
  IlA/1 -> MATLAB Function4/1(Mat)
  MATLAB Function4/1(I11) -> Mux/10
  MATLAB Function4/2(I12) -> Mux/11
  MATLAB Function4/3(I13) -> Mux/12
  MATLAB Function4/5(I22) -> Mux/13
  MATLAB Function4/6(I23) -> Mux/14
  MATLAB Function4/9(I33) -> Mux/15
  MATLAB Function4/4(I21) -> Terminator18/1
  MATLAB Function4/7(I31) -> Terminator19/1
  MATLAB Function4/8(I32) -> Terminator20/1
  MATLAB Function5/8(I32) -> Terminator23/1
  MATLAB Function5/7(I31) -> Terminator22/1
  MATLAB Function5/3(I13) -> Mux/18
  MATLAB Function5/5(I22) -> Mux/19
  MATLAB Function5/4(I21) -> Terminator21/1
  MATLAB Function5/9(I33) -> Mux/21
  MATLAB Function5/1(I11) -> Mux/16
  IlB/1 -> MATLAB Function5/1(Mat)
  MATLAB Function5/2(I12) -> Mux/17
  MATLAB Function5/6(I23) -> Mux/20
  MATLAB Function6/8(I32) -> Terminator26/1
  MATLAB Function6/7(I31) -> Terminator25/1
  MATLAB Function6/3(I13) -> Mux/24
  MATLAB Function6/5(I22) -> Mux/25
  MATLAB Function6/4(I21) -> Terminator24/1
  MATLAB Function6/9(I33) -> Mux/27
  MATLAB Function6/1(I11) -> Mux/22
  IlC/1 -> MATLAB Function6/1(Mat)
  MATLAB Function6/2(I12) -> Mux/23
  MATLAB Function6/6(I23) -> Mux/26
  Demux9/3 -> Mux/45
  Demux9/2 -> Mux/44
  Demux6/3 -> Mux/36
  Demux9/1 -> Mux/43
  Demux6/2 -> Mux/35
  Demux7/1 -> Mux/37
  elA/1 -> Demux8/1
  Constant1/1 -> Mux/59
  elB/1 -> Demux9/1
  Demux8/1 -> Mux/40
  Demux7/2 -> Mux/38
  mlC/1 -> Mux/58
  mlA/1 -> Mux/56
  mLA/1 -> Mux/53
  mLB/1 -> Mux/54
  lB/1 -> Mux/51
  mLC/1 -> Mux/55
  g/1 -> Mux/49
  alphaAB/1 -> Mux/32
  alphaAC/1 -> Mux/33
  elC/1 -> Demux10/1
  mlB/1 -> Mux/57
  Demux10/1 -> Mux/46
  Demux10/2 -> Mux/47
  Demux10/3 -> Mux/48
  Demux7/3 -> Mux/39
  Demux6/1 -> Mux/34
  lC/1 -> Mux/52
  Demux8/2 -> Mux/41
  Constant/1 -> Mux/31
  dq/1 -> Demux7/1
  lA/1 -> Mux/50
  ddq/1 -> Demux6/1
  Demux8/3 -> Mux/42
  LC/1 -> Mux/30
  Demux11/2 -> Mux/61
  Demux11/1 -> Mux/60
  Demux11/3 -> Mux/62
  q/1 -> Demux11/1

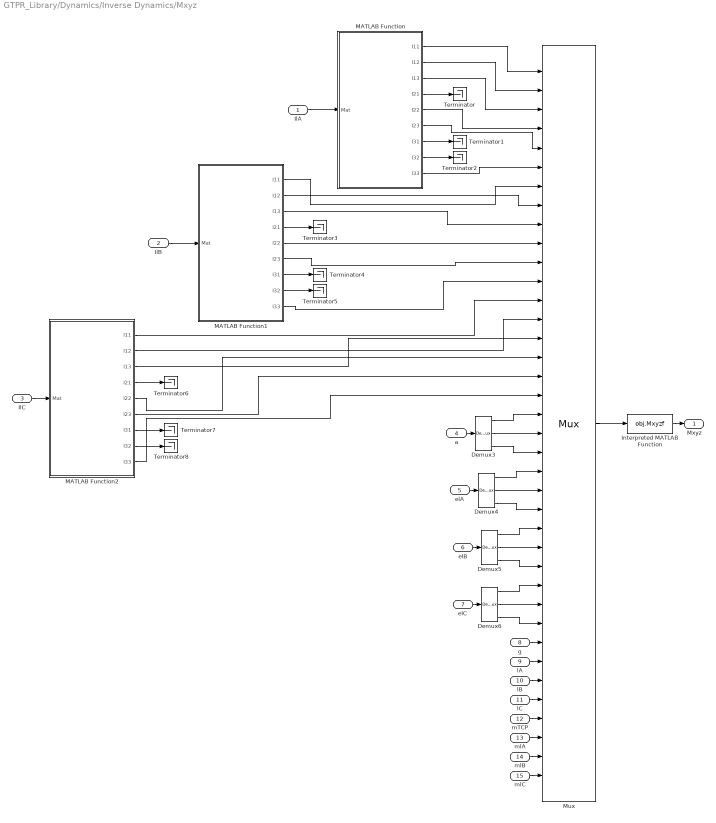
== system GTPR_Library/Dynamics/Inverse Dynamics/Mxyz ==
  IlA : Inport
  IlB : Inport  Port=2
  IlC : Inport  Port=3
  a : Inport  Port=4
  elA : Inport  Port=5
  elB : Inport  Port=6
  elC : Inport  Port=7
  g : Inport  Port=8
  lA : Inport  Port=9
  lB : Inport  Port=10
  lC : Inport  Port=11
  mTCP : Inport  Port=12
  mlA : Inport  Port=13
  mlB : Inport  Port=14
  mlC : Inport  Port=15
  Demux{3..6} (4 alike) : Demux  Outputs=3
  Interpreted MATLAB Function : MATLABFcn  MATLABFcn=obj.Mxyzf
  MATLAB Function : MATLAB Function  TreatAsAtomicUnit=on
  MATLAB Function1 : MATLAB Function  TreatAsAtomicUnit=on
  MATLAB Function2 : MATLAB Function  TreatAsAtomicUnit=on
  Mux : Mux  Inputs=38
  Terminator{,1..8} (9 alike) : Terminator
  Mxyz : Outport
  wires:
  Interpreted MATLAB Function/1 -> Mxyz/1
  Mux/1 -> Interpreted MATLAB Function/1
  a/1 -> Demux3/1
  MATLAB Function/1(I11) -> Mux/1
  mlB/1 -> Mux/37
  mlA/1 -> Mux/36
  lA/1 -> Mux/32
  mlC/1 -> Mux/38
  lC/1 -> Mux/34
  g/1 -> Mux/31
  lB/1 -> Mux/33
  mTCP/1 -> Mux/35
  IlA/1 -> MATLAB Function/1(Mat)
  MATLAB Function/2(I12) -> Mux/2
  MATLAB Function/3(I13) -> Mux/3
  MATLAB Function/5(I22) -> Mux/4
  MATLAB Function/6(I23) -> Mux/5
  MATLAB Function/9(I33) -> Mux/6
  MATLAB Function/4(I21) -> Terminator/1
  MATLAB Function/7(I31) -> Terminator1/1
  MATLAB Function/8(I32) -> Terminator2/1
  MATLAB Function1/4(I21) -> Terminator3/1
  MATLAB Function1/5(I22) -> Mux/10
  MATLAB Function1/6(I23) -> Mux/11
  MATLAB Function1/8(I32) -> Terminator5/1
  MATLAB Function1/1(I11) -> Mux/7
  MATLAB Function1/2(I12) -> Mux/8
  IlB/1 -> MATLAB Function1/1(Mat)
  MATLAB Function1/3(I13) -> Mux/9
  MATLAB Function1/7(I31) -> Terminator4/1
  MATLAB Function1/9(I33) -> Mux/12
  MATLAB Function2/4(I21) -> Terminator6/1
  MATLAB Function2/5(I22) -> Mux/16
  MATLAB Function2/6(I23) -> Mux/17
  MATLAB Function2/8(I32) -> Terminator8/1
  MATLAB Function2/1(I11) -> Mux/13
  MATLAB Function2/2(I12) -> Mux/14
  IlC/1 -> MATLAB Function2/1(Mat)
  MATLAB Function2/3(I13) -> Mux/15
  MATLAB Function2/7(I31) -> Terminator7/1
  MATLAB Function2/9(I33) -> Mux/18
  Demux3/2 -> Mux/20
  Demux3/3 -> Mux/21
  Demux3/1 -> Mux/19
  Demux4/3 -> Mux/24
  Demux4/2 -> Mux/23
  elA/1 -> Demux4/1
  Demux4/1 -> Mux/22
  Demux5/3 -> Mux/27
  Demux5/1 -> Mux/25
  Demux5/2 -> Mux/26
  elB/1 -> Demux5/1
  Demux6/3 -> Mux/30
  Demux6/1 -> Mux/28
  Demux6/2 -> Mux/29
  elC/1 -> Demux6/1

== system GTPR_Library/Dynamics/Inverse Dynamics/dGammaXdqX ==
  LX : Inport
  aX : Inport  Port=2
  alpha : Inport  Port=3
  eX : Inport  Port=4
  qX : Inport  Port=5
  TCP : Inport  Port=6
  Demux : Demux  Outputs=3
  Interpreted MATLAB Function : MATLABFcn  MATLABFcn=obj.dGammaAdq1f
  Mux : Mux  Inputs=8
  dGammaXdqX : Outport
  wires:
  Mux/1 -> Interpreted MATLAB Function/1
  qX/1 -> Mux/5
  LX/1 -> Mux/1
  eX/1 -> Mux/4
  alpha/1 -> Mux/3
  Interpreted MATLAB Function/1 -> dGammaXdqX/1
  aX/1 -> Mux/2
  Demux/2 -> Mux/7
  Demux/1 -> Mux/6
  Demux/3 -> Mux/8
  TCP/1 -> Demux/1

== system GTPR_Library/Dynamics/Inverse Dynamics/elX ==
  LX : Inport
  aX : Inport  Port=2
  alpha : Inport  Port=3
  eX : Inport  Port=4
  qX : Inport  Port=5
  TCP : Inport  Port=6
  Demux : Demux  Outputs=3
  Interpreted MATLAB Function : MATLABFcn  MATLABFcn=obj.elAf(u(1),u(2),u(3),u(4),u(5),u(6:end))  OutputDimensions=3
  Mux : Mux  Inputs=8
  elX : Outport
  wires:
  Interpreted MATLAB Function/1 -> elX/1
  Mux/1 -> Interpreted MATLAB Function/1
  eX/1 -> Mux/4
  aX/1 -> Mux/2
  LX/1 -> Mux/1
  alpha/1 -> Mux/3
  TCP/1 -> Demux/1
  Demux/2 -> Mux/7
  Demux/3 -> Mux/8
  Demux/1 -> Mux/6
  qX/1 -> Mux/5

== system GTPR_Library/Other Functions/Three Spheres Intersection/If Action Subsystem ==
  c1 : Inport
  c2 : Inport  Port=2
  c3 : Inport  Port=3
  r1 : Inport  Port=4
  r2 : Inport  Port=5
  r3 : Inport  Port=6
  Action Port : ActionPort  ActionPortLabel="if(u1 == u2  & u2 == u3)"
  Simplified - ThreeSpheresIntersection : MATLAB Function  TreatAsAtomicUnit=on
  upperIntersection : Outport
  lowerIntersection : Outport  Port=2
  wires:
  Simplified - ThreeSpheresIntersection/2(lowerIntersection) -> lowerIntersection/1
  Simplified - ThreeSpheresIntersection/1(upperIntersection) -> upperIntersection/1
  c1/1 -> Simplified - ThreeSpheresIntersection/1(c1)
  c2/1 -> Simplified - ThreeSpheresIntersection/2(c2)
  c3/1 -> Simplified - ThreeSpheresIntersection/3(c3)
  r1/1 -> Simplified - ThreeSpheresIntersection/4(r1)
  r2/1 -> Simplified - ThreeSpheresIntersection/5(r2)
  r3/1 -> Simplified - ThreeSpheresIntersection/6(r3)

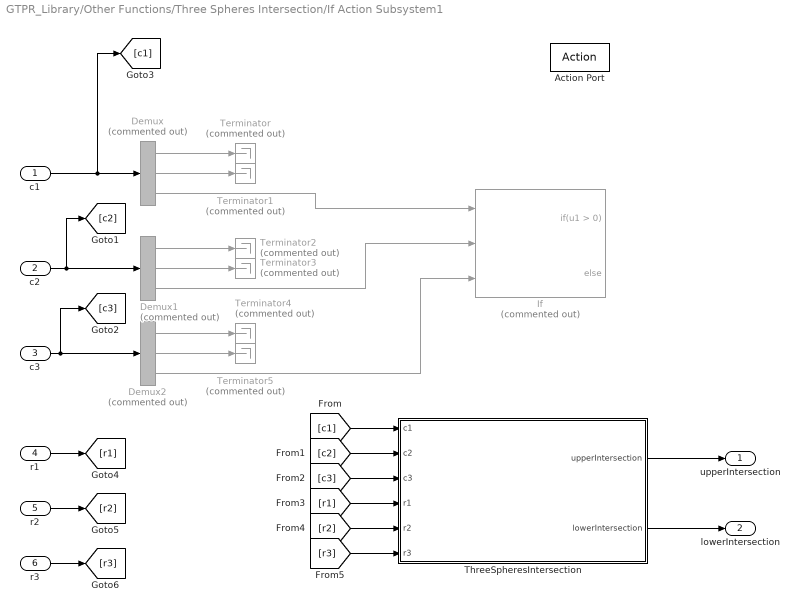
== system GTPR_Library/Other Functions/Three Spheres Intersection/If Action Subsystem1 ==
  c1 : Inport
  c2 : Inport  Port=2
  c3 : Inport  Port=3
  r1 : Inport  Port=4
  r2 : Inport  Port=5
  r3 : Inport  Port=6
  Action Port : ActionPort  ActionPortLabel=else
  Demux : Demux  Commented=on  Outputs=3
  Demux1 : Demux  Commented=on  Outputs=3
  Demux2 : Demux  Commented=on  Outputs=3
  If : If  Commented=on  NumInputs=3
  Terminator{,1..5} (6 alike) : Terminator  Commented=on
  ThreeSpheresIntersection : MATLAB Function  TreatAsAtomicUnit=on
  upperIntersection : Outport
  lowerIntersection : Outport  Port=2
  wires:
  ThreeSpheresIntersection/2(lowerIntersection) -> lowerIntersection/1
  ThreeSpheresIntersection/1(upperIntersection) -> upperIntersection/1
  Demux2/2 -> Terminator5/1
  Demux/2 -> Terminator1/1
  Demux1/2 -> Terminator3/1
  Demux2/1 -> Terminator4/1
  Demux/1 -> Terminator/1
  c2/1 -> [c2], Demux1/1
  Demux2/3 -> If/3
  Demux1/1 -> Terminator2/1
  Demux/3 -> If/1
  c3/1 -> [c3], Demux2/1
  Demux1/3 -> If/2
  c1/1 -> [c1], Demux/1
  r2/1 -> [r2]
  r1/1 -> [r1]
  r3/1 -> [r3]
  [c1] -> ThreeSpheresIntersection/1(c1)
  [c2] -> ThreeSpheresIntersection/2(c2)
  [c3] -> ThreeSpheresIntersection/3(c3)
  [r1] -> ThreeSpheresIntersection/4(r1)
  [r2] -> ThreeSpheresIntersection/5(r2)
  [r3] -> ThreeSpheresIntersection/6(r3)

== matlab function GTPR_Library/Other Functions/Three Spheres Intersection/If Action Subsystem1/ThreeSpheresIntersection ==
  data: c1 input; upperIntersection output; c2 input; c3 input; r1 input; r2 input; r3 input; lowerIntersection output
function [upperIntersection, lowerIntersection] = threeSpheresIntersectionAlgorithm(c1, c2, c3, r1, r2, r3)
    % Three-speheres intersection algorithm from:
    % The Delta Parallel Robot: Kinematics Solutions
    % Robert L. Williams II, Ph.D., williar4@ohio.edu
    % Mechanical Engineering, Ohio University, October 2016
    % Appendix A.

    x1 = c1(1);
    y1 = c1(2);
    z1 = c1(3);

    x2 = c2(1);
    y2 = c2(2);
    z2 = c2(3);

    x3 = c3(1);
    y3 = c3(2);
    z3 = c3(3);


    a11 = 2*(x3-x1);
    a12 = 2*(y3-y1);
    a13 = 2*(z3-z1);

    a21 = 2*(x3-x2);
    a22 = 2*(y3-y2);
    a23 = 2*(z3-z2);

    b1 = power(r1,2)-power(r3,2)-power(x1,2)-power(y1,2)-power(z1,2)+power(x3,2)+power(y3,2)+power(z3,2);
    b2 = power(r2,2)-power(r3,2)-power(x2,2)-power(y2,2)-power(z2,2)+power(x3,2)+power(y3,2)+power(z3,2);

    aA = (a11./a13)-(a21./a23); 
    aB = (a12./a13)-(a22./a23); 
    aC = (b2./a23)-(b1./a13); 
    a4 = -(aB./aA); 
    a5 = -(aC./aA); 
    a6 = (-a21.*a4-a22)./a23;
    a7 = (b2-a21.*a5)./a23;


    a = power(a4,2) + 1 + power(a6,2);
    b = 2.*a4.*(a5-x1)-2.*y1+2.*a6.*(a7-z1);
    c = a5.*(a5-2.*x1)+a7.*(a7-2.*z1)+power(x1,2)+power(y1,2)+power(z1,2)-power(r1,2);



    y = roots([a,b,c]);

    if size(y,2) ~= 2
        y = y';
    end

    x = a4.*y+a5;

    z = a6.*y+a7;
    
    [rows, ~] = find(z(:,2) > z(:,1));

    temp = z(rows,2);
    z(rows,2) = z(rows,1);
    z(rows,1) = temp;

    temp = x(rows,2);
    x(rows,2) = x(rows,1);
    x(rows,1) = temp;

    temp = y(rows,2);
    y(rows,2) = y(rows,1);
    y(rows,1) = temp;

    upperIntersection = [x(1), y(1), z(1)];
    lowerIntersection = [x(2), y(2), z(2)];

== matlab function GTPR_Library/Other Functions/TCP X3/Rz ==
  data: theta input; R output
function R = Rz(theta)

R = [cos(theta), -sin(theta), 0; sin(theta), cos(theta), 0; 0,0,1];

== matlab function GTPR_Library/Other Functions/normalToPlane ==
  data: X1 input; nUnit output; LX input
function nUnit = normalToPlane(X1, LX)

O = [0;0;0];
            
nUnit = cross(O-X1, X1-[0;0;LX]);
nUnit = nUnit / norm(nUnit);

end

    function data = sphereCircleIntersection(cc, rc, nUnit, cs, rs)

    if size(cc) ~= [3,1] %#ok<BDSCA>
        cc = cc';
    end

    if size(cs) ~= [3,1] %#ok<BDSCA>
        cs = cs';
    end

    if size(nUnit) ~= [3,1] %#ok<BDSCA>
        nUnit = nUnit';
    end

    d = dot(nUnit, cc-cs);

    if abs(d) > rs
        data = [];
        return % no intersection
    end

    cp = cs + d*nUnit;

    rp = sqrt(rs^2 - d^2);

    % now the circle circle intersection can be introduced
    dc = norm(cc - cp);

    h = 0.5 + ((rc^2-rp^2)/(2*dc^2));

    ci = cc + h*(cc-cp);

    ri = sqrt(rc^2 - h^2*dc^2);

    % ni = (cc - cp)/d;

    t = cross(cp-cc,nUnit)/norm(cross(cp-cc,nUnit));

    p0 = cc - t*ri + (cc-ci); % Added part for compensation and ci has been modified to cc in both cases
    p1 = cc + t*ri + (cc-ci);

    data.ci = ci;
    data.p0 = p0;
    data.p1 = p1;

    % hold on;
    % plot3(cc(1), cc(2), cc(3), 'bo');
    % quiver3(cc(1), cc(2), cc(3), nUnit(1), nUnit(2), nUnit(3), 'm')
    % 
    % plot3(cs(1), cs(2), cs(3), 'bs');
    % 
    % plot3(ci(1), ci(2), ci(3), 'ro');
    % plot3(p0(1), p0(2), p0(3), 'rx');
    % plot3(p1(1), p1(2), p1(3), 'r*');

    end

== matlab function GTPR_Library/Other Functions/sphereCircleIntersection ==
  data: cc input; p0 output; rc input; nUnit input; cs input; rs input
function p0 = sphereCircleIntersection(cc, rc, nUnit, cs, rs)
%https://gamedev.stackexchange.com/questions/75756/sphere-sphere-intersection-and-circle-sphere-intersection
    if size(cc) ~= [3,1] %#ok<BDSCA>
        cc = cc';
    end

    if size(cs) ~= [3,1] %#ok<BDSCA>
        cs = cs';
    end

    if size(nUnit) ~= [3,1] %#ok<BDSCA>
        nUnit = nUnit';
    end

    d = dot(nUnit, cc-cs);

    if abs(d) > rs
%         data = [];
        p0 = [];
        return % no intersection
    end

    cp = cs + d*nUnit;

    rp = sqrt(rs^2 - d^2);

    % now the circle circle intersection can be introduced
    dc = norm(cc - cp);

    h = 0.5 + ((rc^2-rp^2)/(2*dc^2));

    ci = cc + h*(cc-cp);

    ri = sqrt(rc^2 - h^2*dc^2);

    % ni = (cc - cp)/d;

    t = cross(cp-cc,nUnit)/norm(cross(cp-cc,nUnit));

    p0 = cc - t*ri + (cc-ci); % Added part for compensation and ci has been modified to cc in both cases
%     p1 = cc + t*ri + (cc-ci);

%     data.ci = ci;
%     data.p0 = p0;
%     data.p1 = p1;

end

== matlab function GTPR_Library/Geometry/Inverse Geometry/normalToPlane ==
  data: X1 input; nUnit output size=[3 1]; LX input
function nUnit = normalToPlane(X1, LX)

O = [0;0;0];
            
nUnit = cross(O-X1, X1-[0;0;LX]);
nUnit = nUnit / norm(nUnit);

end

    function data = sphereCircleIntersection(cc, rc, nUnit, cs, rs)

    if size(cc) ~= [3,1] %#ok<BDSCA>
        cc = cc';
    end

    if size(cs) ~= [3,1] %#ok<BDSCA>
        cs = cs';
    end

    if size(nUnit) ~= [3,1] %#ok<BDSCA>
        nUnit = nUnit';
    end

    d = dot(nUnit, cc-cs);

    if abs(d) > rs
        data = [];
        return % no intersection
    end

    cp = cs + d*nUnit;

    rp = sqrt(rs^2 - d^2);

    % now the circle circle intersection can be introduced
    dc = norm(cc - cp);

    h = 0.5 + ((rc^2-rp^2)/(2*dc^2));

    ci = cc + h*(cc-cp);

    ri = sqrt(rc^2 - h^2*dc^2);

    % ni = (cc - cp)/d;

    t = cross(cp-cc,nUnit)/norm(cross(cp-cc,nUnit));

    p0 = cc - t*ri + (cc-ci); % Added part for compensation and ci has been modified to cc in both cases
    p1 = cc + t*ri + (cc-ci);

    data.ci = ci;
    data.p0 = p0;
    data.p1 = p1;

    % hold on;
    % plot3(cc(1), cc(2), cc(3), 'bo');
    % quiver3(cc(1), cc(2), cc(3), nUnit(1), nUnit(2), nUnit(3), 'm')
    % 
    % plot3(cs(1), cs(2), cs(3), 'bs');
    % 
    % plot3(ci(1), ci(2), ci(3), 'ro');
    % plot3(p0(1), p0(2), p0(3), 'rx');
    % plot3(p1(1), p1(2), p1(3), 'r*');

    end

== matlab function GTPR_Library/Geometry/Inverse Geometry/normalToPlane1 ==
  data: X1 input; nUnit output size=[3 1]; LX input
function nUnit = normalToPlane(X1, LX)

O = [0;0;0];
            
nUnit = cross(O-X1, X1-[0;0;LX]);
nUnit = nUnit / norm(nUnit);

end

    function data = sphereCircleIntersection(cc, rc, nUnit, cs, rs)

    if size(cc) ~= [3,1] %#ok<BDSCA>
        cc = cc';
    end

    if size(cs) ~= [3,1] %#ok<BDSCA>
        cs = cs';
    end

    if size(nUnit) ~= [3,1] %#ok<BDSCA>
        nUnit = nUnit';
    end

    d = dot(nUnit, cc-cs);

    if abs(d) > rs
        data = [];
        return % no intersection
    end

    cp = cs + d*nUnit;

    rp = sqrt(rs^2 - d^2);

    % now the circle circle intersection can be introduced
    dc = norm(cc - cp);

    h = 0.5 + ((rc^2-rp^2)/(2*dc^2));

    ci = cc + h*(cc-cp);

    ri = sqrt(rc^2 - h^2*dc^2);

    % ni = (cc - cp)/d;

    t = cross(cp-cc,nUnit)/norm(cross(cp-cc,nUnit));

    p0 = cc - t*ri + (cc-ci); % Added part for compensation and ci has been modified to cc in both cases
    p1 = cc + t*ri + (cc-ci);

    data.ci = ci;
    data.p0 = p0;
    data.p1 = p1;

    % hold on;
    % plot3(cc(1), cc(2), cc(3), 'bo');
    % quiver3(cc(1), cc(2), cc(3), nUnit(1), nUnit(2), nUnit(3), 'm')
    % 
    % plot3(cs(1), cs(2), cs(3), 'bs');
    % 
    % plot3(ci(1), ci(2), ci(3), 'ro');
    % plot3(p0(1), p0(2), p0(3), 'rx');
    % plot3(p1(1), p1(2), p1(3), 'r*');

    end
